simulink model "Part2_DynamicsModel"  (R2016a)
settings: Solver=VariableStepAuto  StartTime=0.0  StopTime=10.0  RelTol=1e-3
settings Model: Creator=Farhan  LastModifiedBy=Farhan

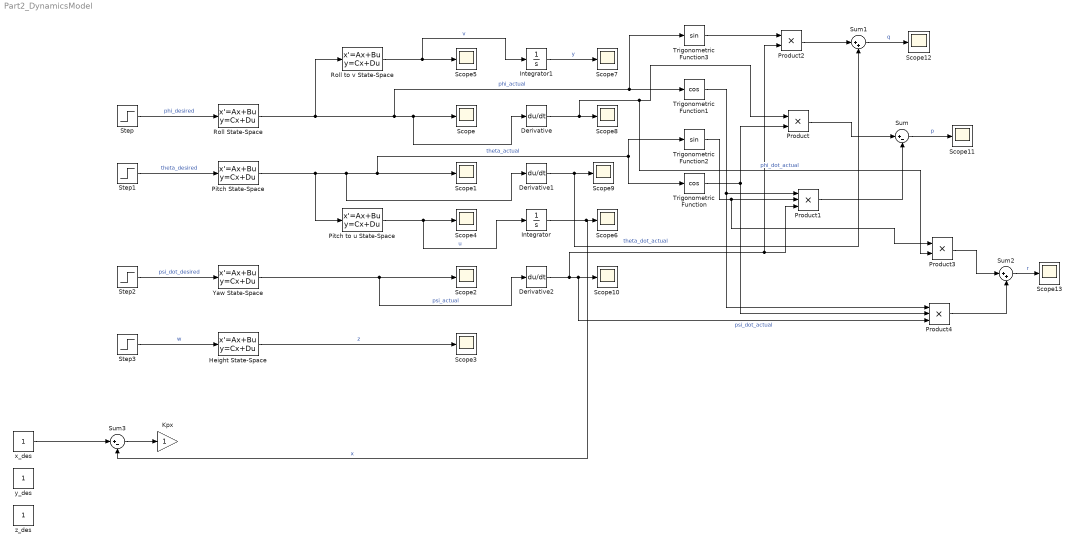
== system Part2_DynamicsModel ==
  Derivative : Derivative
  Derivative1 : Derivative
  Derivative2 : Derivative
  Height State-Space : StateSpace  A=[-5.82 -3.6046*exp(1)^-6; 3.8147*exp(1)^-6 0]  B=[1024; 0]  C=[1.4907*exp(1)^-4 1.3191*exp(1)^3]  D=0  X0=0  ContinuousStateAttributes='Height'
  Integrator : Integrator
  Integrator1 : Integrator
  Kpx : Gain
  Pitch State-Space : StateSpace  A=[-3.9784 -2.9796; 4 0]  B=[2; 0]  C=[1.2569 0.6083]  D=0  X0=0  ContinuousStateAttributes='Pitch'
  Pitch to u State-Space : StateSpace  A=-0.665  B=2  C=-3.0772  D=0  X0=0  ContinuousStateAttributes='Pitch_to_u'
  Product : Product
  Product1 : Product  Inputs=3
  Product2 : Product
  Product3 : Product
  Product4 : Product  Inputs=3
  Roll State-Space : StateSpace  A=[-4.2683 -3.1716; 4 0]  B=[2; 0]  C=[0.7417 0.4405]  D=0  X0=0  ContinuousStateAttributes='Roll'
  Roll to v State-Space : StateSpace  A=-0.4596  B=2  C=2.3868  D=0  X0=0  ContinuousStateAttributes='Roll_to_v'
  Scope{,1..13} (14 alike) : Scope
  Step{,1..3} (4 alike) : Step  SampleTime=0
  Sum : Sum  Inputs=|+-
  Sum1 : Sum  Inputs=|++
  Sum2 : Sum  Inputs=|++
  Sum3 : Sum  Inputs=|+-
  Trigonometric Function : Trigonometry  Operator=cos
  Trigonometric Function1 : Trigonometry  Operator=cos
  Trigonometric Function2 : Trigonometry
  Trigonometric Function3 : Trigonometry
  Yaw State-Space : StateSpace  A=-0.0059  C=1.2653  D=0  X0=0  ContinuousStateAttributes='Yaw'
  x_des : Constant
  y_des : Constant
  z_des : Constant
  wires:
  Step/1 -> Roll State-Space/1  "phi_desired"
  Roll State-Space/1 -> Roll to v State-Space/1, Trigonometric Function3/1, Trigonometric Function1/1, Derivative/1, Scope/1  "phi_actual"
  Step1/1 -> Pitch State-Space/1  "theta_desired"
  Pitch State-Space/1 -> Pitch to u State-Space/1, Derivative1/1, Trigonometric Function2/1, Trigonometric Function/1, Scope1/1  "theta_actual"
  Step2/1 -> Yaw State-Space/1  "psi_dot_desired"
  Yaw State-Space/1 -> Derivative2/1, Scope2/1  "psi_actual"
  Step3/1 -> Height State-Space/1  "w"
  Height State-Space/1 -> Scope3/1  "z"
  Pitch to u State-Space/1 -> Integrator/1, Scope4/1  "u"
  Roll to v State-Space/1 -> Integrator1/1, Scope5/1  "v"
  Integrator/1 -> Sum3/2, Scope6/1  "x"
  Integrator1/1 -> Scope7/1  "y"
  Derivative/1 -> Product3/2, Product/1, Scope8/1  "phi_dot_actual"
  Derivative1/1 -> Sum1/2, Scope9/1  "theta_dot_actual"
  Derivative2/1 -> Product2/2, Product1/3, Product4/3, Scope10/1  "psi_dot_actual"
  Trigonometric Function/1 -> Product/2, Product4/2
  Trigonometric Function1/1 -> Product4/1, Product1/1
  Trigonometric Function2/1 -> Product3/1, Product1/2
  Product/1 -> Sum/1
  Product1/1 -> Sum/2
  Sum/1 -> Scope11/1  "p"
  Trigonometric Function3/1 -> Product2/1
  Product2/1 -> Sum1/1
  Sum1/1 -> Scope12/1  "q"
  Product3/1 -> Sum2/1
  Product4/1 -> Sum2/2
  Sum2/1 -> Scope13/1  "r"
  x_des/1 -> Sum3/1
  Sum3/1 -> Kpx/1
